simulink model "Motor_DC"  (R2024a)
settings: Solver=VariableStepAuto  StartTime=0.0  StopTime=1  RelTol=1e-3
settings Model: Creator=adobe  LastModifiedBy=adobe

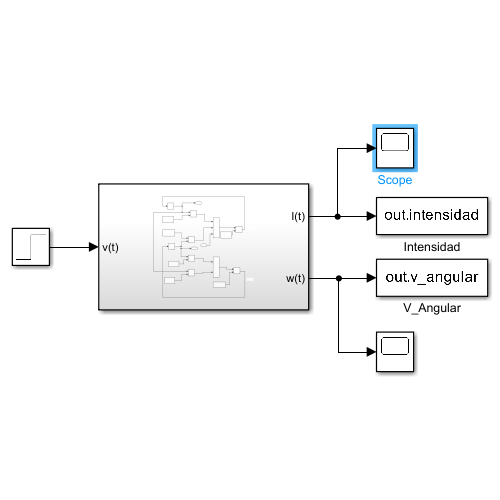
[thumbnail: Simulink's stored preview of the top-level diagram]
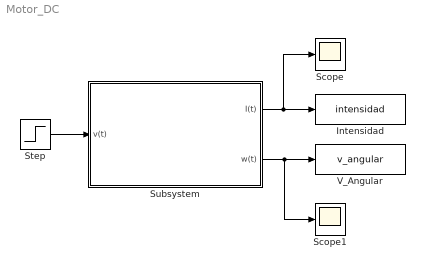
== system Motor_DC ==
  Intensidad : ToWorkspace  VariableName=intensidad  SampleTime=-1
  Scope : Scope
  Scope1 : Scope
  Step : Step  Time=0.5  After=10.5  SampleTime=0
  Subsystem : Subsystem
  V_Angular : ToWorkspace  VariableName=v_angular  SampleTime=-1
  wires:
  Step/1 -> Subsystem/1(v(t))
  Subsystem/1(I(t)) -> Scope/1, Intensidad/1
  Subsystem/2(w(t)) -> Scope1/1, V_Angular/1

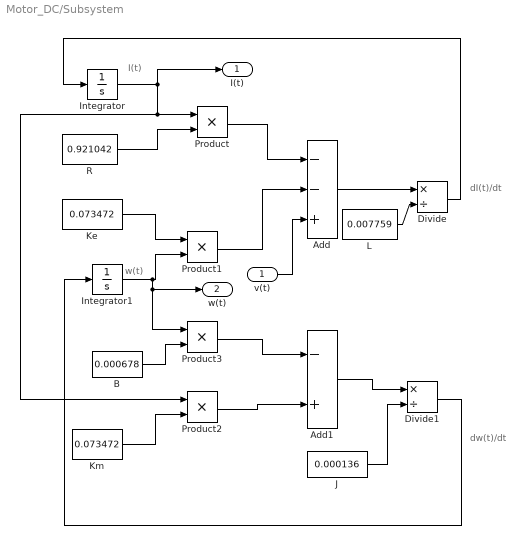
== system Motor_DC/Subsystem ==
  note: w(t)
  note: I(t)
  note: dI(t)/dt
  note: dw(t)/dt
  v(t) : Inport
  Add : Sum  Inputs=--+
  Add1 : Sum  Inputs=-+
  B : Constant  Value=0.000678
  Divide : Product  Inputs=*/
  Divide1 : Product  Inputs=*/
  Integrator : Integrator
  Integrator1 : Integrator
  J : Constant  Value=0.000136
  Ke : Constant  Value=0.073472
  Km : Constant  Value=0.073472
  L : Constant  Value=0.007759
  Product{,1..3} (4 alike) : Product
  R : Constant  Value=0.921042
  I(t) : Outport
  w(t) : Outport  Port=2
  wires:
  Divide1/1 -> Integrator1/1
  Add1/1 -> Divide1/1
  L/1 -> Divide/2
  Ke/1 -> Product1/1
  Product3/1 -> Add1/1
  v(t)/1 -> Add/3
  Integrator1/1 -> w(t)/1, Product3/1, Product1/2
  Integrator/1 -> I(t)/1, Product2/1, Product/1
  J/1 -> Divide1/2
  Add/1 -> Divide/1
  Km/1 -> Product2/2
  Product2/1 -> Add1/2
  R/1 -> Product/2
  Divide/1 -> Integrator/1
  Product1/1 -> Add/2
  B/1 -> Product3/2
  Product/1 -> Add/1
